simulink model "usv_twist_controller_generator_002"  (R2021b)
settings: Solver=FixedStepDiscrete  StartTime=0.0  StopTime=inf  FixedStep=twistControllerSampleTime  RelTol=1e-3  EnableMultiTasking=on
PreLoadFcn:
  | % Controller Sample Time
  | twistControllerSampleTime = 0.10;
undefined symbols (not defined in the file): DiscIntNeverNeededParam
libraries: robotlib x28, simulink x4
settings Model: Creator=altin  LastModifiedBy=altin
settings SolverCC: AllowMultiTaskInputOutput=on  ConcurrentTasks=on  PositivePriorityOrder=on  AutoInsertRateTranBlk=on
settings OptimizationCC: EnhancedBackFolding=on  PassReuseOutputArgsAs=Individual arguments  ZeroExternalMemoryAtStartup=off  ZeroInternalMemoryAtStartup=off  MaxStackSize=64  OptimizeBlockOrder=speed  DifferentSizesBufferReuse=on  OptimizationCustomize=off  EfficientTunableParamExpr=on
settings DebuggingCC: ParameterTunabilityLossMsg=error
settings HardwareCC: ProdBitPerPointer=32  ProdBitPerSizeT=32  ProdBitPerPtrDiffT=32  ProdLargestAtomicFloat=None  ProdIntDivRoundTo=Undefined  ProdEndianess=Unspecified  ProdWordSize=32  ProdHWDeviceType=Generic->Unspecified (assume 32-bit Generic)  UseEmbeddedCoderFeatures=off
settings ModelReferenceCC: ModelReferenceMinAlgLoopOccurrences=on
settings SFSimCC: MATLABDynamicMemAlloc=off
settings RTWCC: Description=Embedded Coder  SystemTargetFile=ert.tlc  HardwareBoard=Robot Operating System (ROS)  TLCOptions="-aInlineSetEventsForThisBaseRateFcn=TLC_FALSE -aSuppressMultiTaskScheduler=TLC_FALSE  -aRateBasedStepFcn=0"  TemplateMakefile=ert_default_tmf  GenerateReport=on  Toolchain=Catkin  LaunchReport=on  TargetLang=C++
settings CodeAppCC: ForceParamTrailComments=on  IgnoreCustomStorageClasses=off  OperatorAnnotations=on  SimulinkDataObjDesc=on  SFDataObjDesc=on  InsertBlockDesc=on  StateflowObjectComments=on  MATLABSourceComments=on
settings ERTTargetCC: SupportNonInlinedSFcns=on  ERTCustomFileTemplate=rostime_codertarget_file_process.tlc

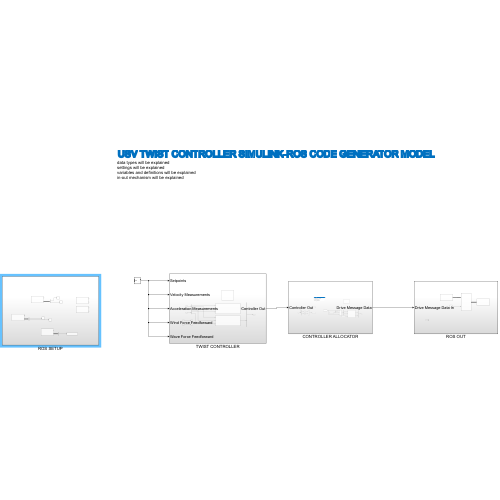
[thumbnail: Simulink's stored preview of the top-level diagram]
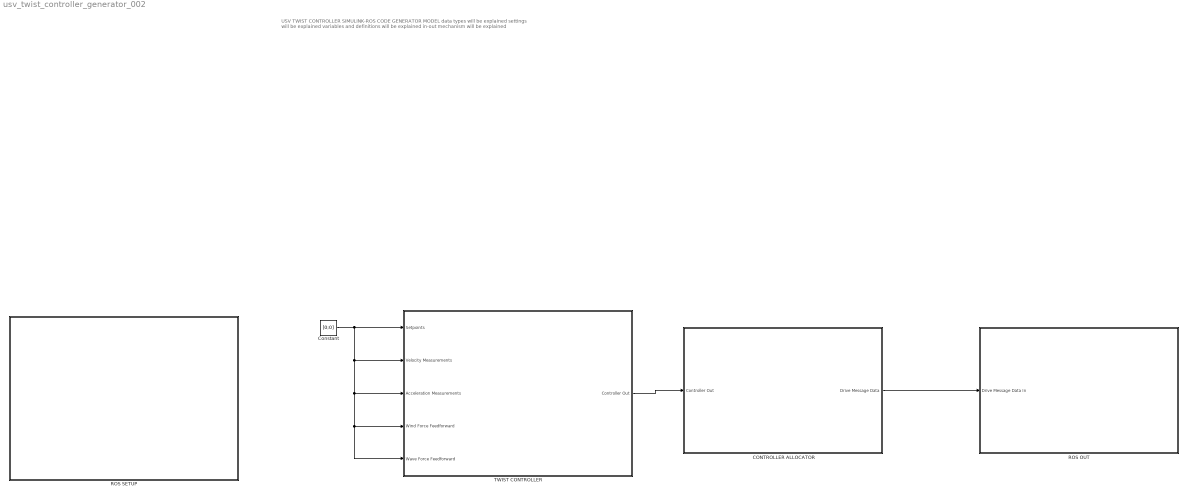
== system usv_twist_controller_generator_002 ==
  note: USV TWIST CONTROLLER SIMULINK-ROS CODE GENERATOR MODEL
      | data types will be explained
      | settings will be explained
      | variables and definitions will be explained
      | in-out mechanism will be explained
  CONTROLLER ALLOCATOR : Subsystem
  Constant : Constant  Value=[0;0]
  ROS OUT : Subsystem
  ROS SETUP : Subsystem
  TWIST CONTROLLER : Subsystem
  wires:
  TWIST CONTROLLER/1(Controller Out) -> CONTROLLER ALLOCATOR/1(Controller Out)
  CONTROLLER ALLOCATOR/1(Drive Message Data) -> ROS OUT/1(Drive Message Data In)
  Constant/1 -> TWIST CONTROLLER/1(Setpoints), TWIST CONTROLLER/2(Velocity Measurements), TWIST CONTROLLER/4(Wind Force Feedforward), TWIST CONTROLLER/5(Wave Force Feedforward), TWIST CONTROLLER/3(Acceleration Measurements)

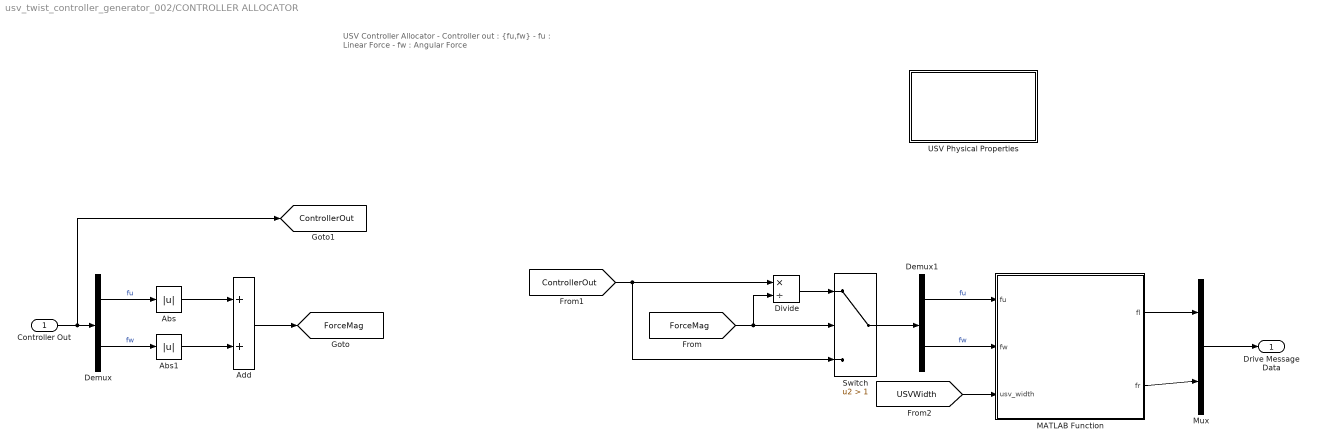
== system usv_twist_controller_generator_002/CONTROLLER ALLOCATOR ==
  note: USV Controller Allocator
      | - Controller out : {fu,fw}
      | - fu : Linear Force
      | - fw : Angular Force
  Controller Out : Inport
  Abs : Abs
  Abs1 : Abs
  Add : Sum
  Demux : Demux  Outputs=2
  Demux1 : Demux  Outputs=2
  Divide : Product  Inputs=*/
  MATLAB Function : MATLAB Function  TreatAsAtomicUnit=on
  Mux : Mux  Inputs=2
  Switch : Switch  Criteria=u2 > Threshold  Threshold=1
  USV Physical Properties : Subsystem
  Drive Message Data : Outport
  tag scope: ControllerOut=global, ForceMag=global
  wires:
  Controller Out/1 -> [ControllerOut], Demux/1
  Demux/1 -> Abs/1  "fu"
  Demux/2 -> Abs1/1  "fw"
  Abs1/1 -> Add/2
  Abs/1 -> Add/1
  Add/1 -> [ForceMag]
  [ForceMag] -> Divide/2, Switch/2
  [ControllerOut] -> Switch/3, Divide/1
  Divide/1 -> Switch/1
  Switch/1 -> Demux1/1
  [USVWidth] -> MATLAB Function/3(usv_width)
  Demux1/1 -> MATLAB Function/1(fu)  "fu"
  Demux1/2 -> MATLAB Function/2(fw)  "fw"
  MATLAB Function/1(fl) -> Mux/1
  MATLAB Function/2(fr) -> Mux/2
  Mux/1 -> Drive Message Data/1

== system usv_twist_controller_generator_002/ROS OUT ==
  Drive Message Data In : Inport
  Bus Assignment : BusAssignment  AssignedSignals=Data
  Constant : Constant  OutDataTypeStr=int32
  Motor Drive Message : robotlib/Blank Message  messageClass=Message  entityType=std_msgs/Int32  messageType=std_msgs/Int32  SampleTime=inf  legacyBusStruct=off
  USV Drive Topic : robotlib/Publish  topicSource=Specify your own  topic=/chatter2  messageType=std_msgs/Int32  legacyBusStruct=off  messageQueueLength=1
  wires:
  Motor Drive Message/1 -> Bus Assignment/1
  Constant/1 -> Bus Assignment/2
  Bus Assignment/1 -> USV Drive Topic/1

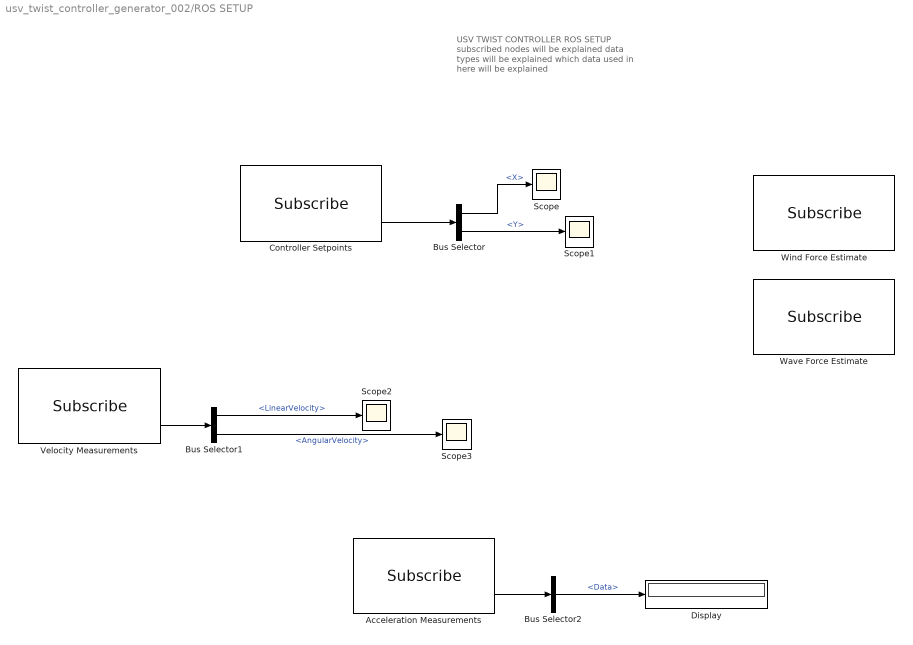
== system usv_twist_controller_generator_002/ROS SETUP ==
  note: USV TWIST CONTROLLER ROS SETUP
      | subscribed nodes will be explained
      | data types will be explained
      | which data used in here will be explained
  Acceleration Measurements : robotlib/Subscribe  topicSource=Select from ROS network  topic=/chatter  messageType=std_msgs/Int32  SampleTime=-1  legacyBusStruct=off  messageQueueLength=1
  Bus Selector : BusSelector  OutputSignals=X,Y
  Bus Selector1 : BusSelector  OutputSignals=LinearVelocity,AngularVelocity
  Bus Selector2 : BusSelector  OutputSignals=Data
  Controller Setpoints : robotlib/Subscribe  topicSource=Specify your own  topic=/gx5/nav/odom  messageType=geometry_msgs/Point  SampleTime=-1  legacyBusStruct=off  messageQueueLength=1
  Display : Display
  Scope{,1..3} (4 alike) : Scope
  Velocity Measurements : robotlib/Subscribe  topicSource=Select from ROS network  topic=/turtle1/pose  messageType=turtlesim/Pose  SampleTime=-1  legacyBusStruct=off  messageQueueLength=1
  Wave Force Estimate : robotlib/Subscribe  topicSource=Select from ROS network  topic=/my_topic  messageType=geometry_msgs/Point  SampleTime=-1  legacyBusStruct=off  messageQueueLength=1
  Wind Force Estimate : robotlib/Subscribe  topicSource=Select from ROS network  topic=/my_topic  messageType=geometry_msgs/Point  SampleTime=-1  legacyBusStruct=off  messageQueueLength=1
  wires:
  Controller Setpoints/2 -> Bus Selector/1
  Bus Selector/1 -> Scope/1  "<X>"
  Bus Selector/2 -> Scope1/1  "<Y>"
  Velocity Measurements/2 -> Bus Selector1/1
  Bus Selector1/1 -> Scope2/1  "<LinearVelocity>"
  Bus Selector1/2 -> Scope3/1  "<AngularVelocity>"
  Acceleration Measurements/2 -> Bus Selector2/1
  Bus Selector2/1 -> Display/1  "<Data>"

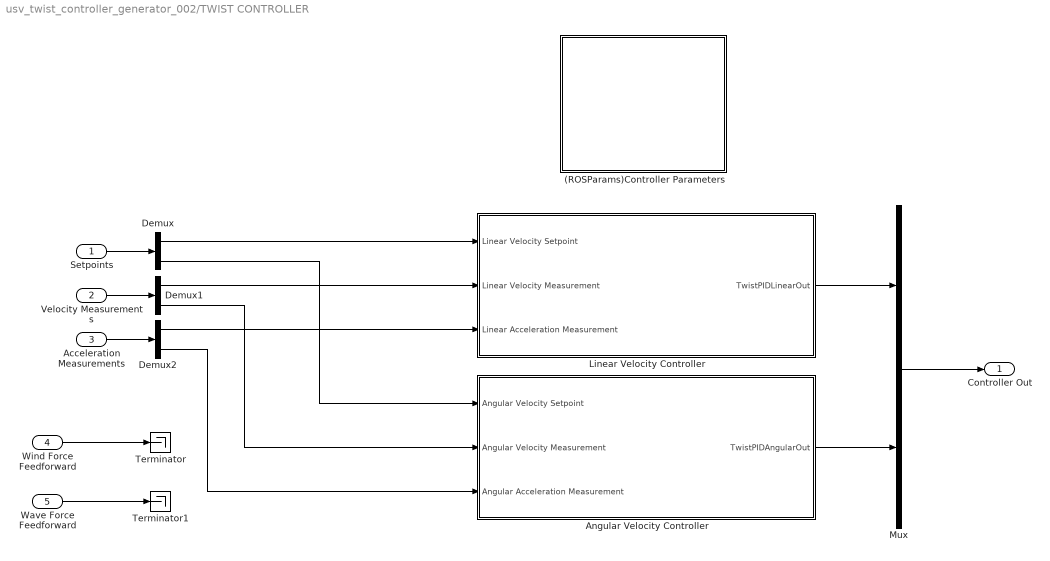
== system usv_twist_controller_generator_002/TWIST CONTROLLER ==
  Setpoints : Inport
  Velocity Measurements : Inport  Port=2
  Acceleration Measurements : Inport  Port=3
  Wind Force Feedforward : Inport  Port=4
  Wave Force Feedforward : Inport  Port=5
  (ROSParams)Controller Parameters : Subsystem
  Angular Velocity Controller : Subsystem
  Demux : Demux  Outputs=2
  Demux1 : Demux  Outputs=2
  Demux2 : Demux  Outputs=2
  Linear Velocity Controller : Subsystem
  Mux : Mux  Inputs=2
  Terminator : Terminator
  Terminator1 : Terminator
  Controller Out : Outport
  wires:
  Setpoints/1 -> Demux/1
  Demux/1 -> Linear Velocity Controller/1(Linear Velocity Setpoint)
  Demux/2 -> Angular Velocity Controller/1(Angular Velocity Setpoint)
  Wind Force Feedforward/1 -> Terminator/1
  Wave Force Feedforward/1 -> Terminator1/1
  Acceleration Measurements/1 -> Demux2/1
  Velocity Measurements/1 -> Demux1/1
  Demux1/1 -> Linear Velocity Controller/2(Linear Velocity Measurement)
  Demux1/2 -> Angular Velocity Controller/2(Angular Velocity Measurement)
  Demux2/1 -> Linear Velocity Controller/3(Linear Acceleration Measurement)
  Demux2/2 -> Angular Velocity Controller/3(Angular Acceleration Measurement)
  Linear Velocity Controller/1(TwistPIDLinearOut) -> Mux/1
  Angular Velocity Controller/1(TwistPIDAngularOut) -> Mux/2
  Mux/1 -> Controller Out/1

== system usv_twist_controller_generator_002/CONTROLLER ALLOCATOR/USV Physical Properties ==
  Twist Angular Ag : robotlib/Get Parameter  ParameterSource=Select from ROS network  ParameterName=/my_param  ParameterType=double  ParameterMaxArrayLength=16  ParameterInitialValue=0.0  SampleTime=-1  ShowErrorCodeOutput=on  ModelName=usv_twist_controller_generator_002  BlockId=ParamGet_usv_twist_controller_generator_002_280
      settings: SourceProductBaseCode=RR
  tag scope: USVWidth=global
  wires:
  Twist Angular Ag/1 -> [USVWidth]

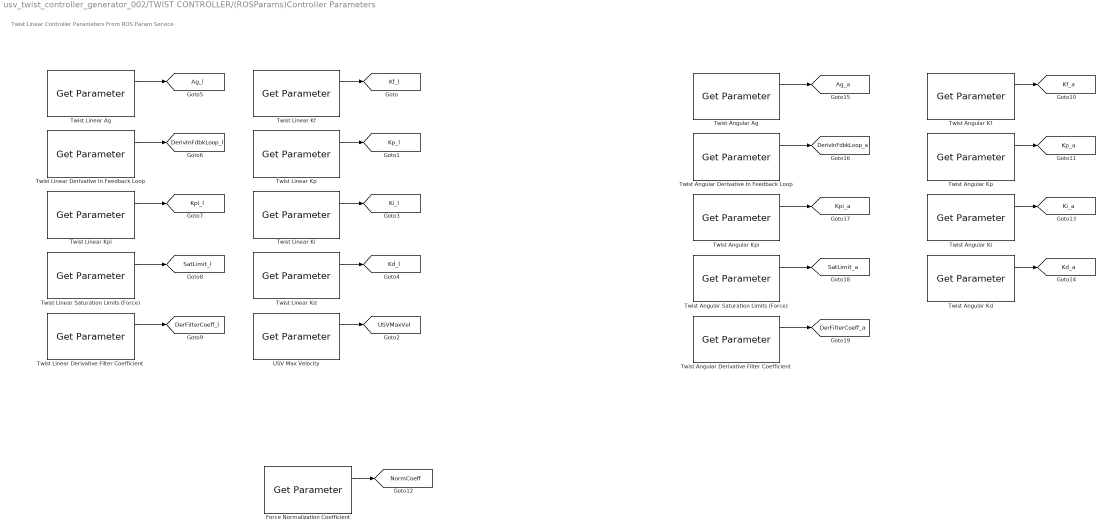
== system usv_twist_controller_generator_002/TWIST CONTROLLER/(ROSParams)Controller Parameters ==
  note: Twist Linear Controller Parameters From ROS Param Service
  Force Normalization Coefficient : robotlib/Get Parameter  ParameterSource=Select from ROS network  ParameterName=/my_param  ParameterType=double  ParameterMaxArrayLength=16  ParameterInitialValue=0.0  SampleTime=-1  ShowErrorCodeOutput=on  ModelName=usv_twist_controller_generator_002  BlockId=ParamGet_usv_twist_controller_generator_002_290
      settings: SourceProductBaseCode=RR
  Twist Angular Ag : robotlib/Get Parameter  ParameterSource=Select from ROS network  ParameterName=/my_param  ParameterType=double  ParameterMaxArrayLength=16  ParameterInitialValue=0.0  SampleTime=-1  ShowErrorCodeOutput=on  ModelName=usv_twist_controller_generator_002  BlockId=ParamGet_usv_twist_controller_generator_002_169
      settings: SourceProductBaseCode=RR
  Twist Angular Derivative Filter Coefficient : robotlib/Get Parameter  ParameterSource=Select from ROS network  ParameterName=/my_param  ParameterType=double  ParameterMaxArrayLength=16  ParameterInitialValue=0.0  SampleTime=-1  ShowErrorCodeOutput=on  ModelName=usv_twist_controller_generator_002  BlockId=ParamGet_usv_twist_controller_generator_002_170
      settings: SourceProductBaseCode=RR
  Twist Angular Derivative In Feedback Loop : robotlib/Get Parameter  ParameterSource=Select from ROS network  ParameterName=/my_param  ParameterType=double  ParameterMaxArrayLength=16  ParameterInitialValue=0.0  SampleTime=-1  ShowErrorCodeOutput=on  ModelName=usv_twist_controller_generator_002  BlockId=ParamGet_usv_twist_controller_generator_002_171
      settings: SourceProductBaseCode=RR
  Twist Angular Kd : robotlib/Get Parameter  ParameterSource=Select from ROS network  ParameterName=/my_param  ParameterType=double  ParameterMaxArrayLength=16  ParameterInitialValue=0.0  SampleTime=-1  ShowErrorCodeOutput=on  ModelName=usv_twist_controller_generator_002  BlockId=ParamGet_usv_twist_controller_generator_002_172
      settings: SourceProductBaseCode=RR
  Twist Angular Kf : robotlib/Get Parameter  ParameterSource=Select from ROS network  ParameterName=/my_param  ParameterType=double  ParameterMaxArrayLength=16  ParameterInitialValue=0.0  SampleTime=-1  ShowErrorCodeOutput=on  ModelName=usv_twist_controller_generator_002  BlockId=ParamGet_usv_twist_controller_generator_002_173
      settings: SourceProductBaseCode=RR
  Twist Angular Ki : robotlib/Get Parameter  ParameterSource=Select from ROS network  ParameterName=/my_param  ParameterType=double  ParameterMaxArrayLength=16  ParameterInitialValue=0.0  SampleTime=-1  ShowErrorCodeOutput=on  ModelName=usv_twist_controller_generator_002  BlockId=ParamGet_usv_twist_controller_generator_002_174
      settings: SourceProductBaseCode=RR
  Twist Angular Kp : robotlib/Get Parameter  ParameterSource=Select from ROS network  ParameterName=/my_param  ParameterType=double  ParameterMaxArrayLength=16  ParameterInitialValue=0.0  SampleTime=-1  ShowErrorCodeOutput=on  ModelName=usv_twist_controller_generator_002  BlockId=ParamGet_usv_twist_controller_generator_002_175
      settings: SourceProductBaseCode=RR
  Twist Angular Kpi : robotlib/Get Parameter  ParameterSource=Select from ROS network  ParameterName=/my_param  ParameterType=double  ParameterMaxArrayLength=16  ParameterInitialValue=0.0  SampleTime=-1  ShowErrorCodeOutput=on  ModelName=usv_twist_controller_generator_002  BlockId=ParamGet_usv_twist_controller_generator_002_176
      settings: SourceProductBaseCode=RR
  Twist Angular Saturation Limits (Force) : robotlib/Get Parameter  ParameterSource=Select from ROS network  ParameterName=/my_param  ParameterType=double  ParameterMaxArrayLength=16  ParameterInitialValue=0.0  SampleTime=-1  ShowErrorCodeOutput=on  ModelName=usv_twist_controller_generator_002  BlockId=ParamGet_usv_twist_controller_generator_002_177
      settings: SourceProductBaseCode=RR
  Twist Linear Ag : robotlib/Get Parameter  ParameterSource=Select from ROS network  ParameterName=/my_param  ParameterType=double  ParameterMaxArrayLength=16  ParameterInitialValue=0.0  SampleTime=-1  ShowErrorCodeOutput=on  ModelName=usv_twist_controller_generator_002  BlockId=ParamGet_usv_twist_controller_generator_002_9
      settings: SourceProductBaseCode=RR
  Twist Linear Derivative Filter Coefficient : robotlib/Get Parameter  ParameterSource=Select from ROS network  ParameterName=/my_param  ParameterType=double  ParameterMaxArrayLength=16  ParameterInitialValue=0.0  SampleTime=-1  ShowErrorCodeOutput=on  ModelName=usv_twist_controller_generator_002  BlockId=ParamGet_usv_twist_controller_generator_002_50
      settings: SourceProductBaseCode=RR
  Twist Linear Derivative In Feedback Loop : robotlib/Get Parameter  ParameterSource=Select from ROS network  ParameterName=/my_param  ParameterType=double  ParameterMaxArrayLength=16  ParameterInitialValue=0.0  SampleTime=-1  ShowErrorCodeOutput=on  ModelName=usv_twist_controller_generator_002  BlockId=ParamGet_usv_twist_controller_generator_002_10
      settings: SourceProductBaseCode=RR
  Twist Linear Kd : robotlib/Get Parameter  ParameterSource=Select from ROS network  ParameterName=/my_param  ParameterType=double  ParameterMaxArrayLength=16  ParameterInitialValue=0.0  SampleTime=-1  ShowErrorCodeOutput=on  ModelName=usv_twist_controller_generator_002  BlockId=ParamGet_usv_twist_controller_generator_002_8
      settings: SourceProductBaseCode=RR
  Twist Linear Kf : robotlib/Get Parameter  ParameterSource=Select from ROS network  ParameterName=/my_param  ParameterType=double  ParameterMaxArrayLength=16  ParameterInitialValue=0.0  SampleTime=-1  ShowErrorCodeOutput=on  ModelName=usv_twist_controller_generator_002  BlockId=ParamGet_usv_twist_controller_generator_002_11
      settings: SourceProductBaseCode=RR
  Twist Linear Ki : robotlib/Get Parameter  ParameterSource=Select from ROS network  ParameterName=/my_param  ParameterType=double  ParameterMaxArrayLength=16  ParameterInitialValue=0.0  SampleTime=-1  ShowErrorCodeOutput=on  ModelName=usv_twist_controller_generator_002  BlockId=ParamGet_usv_twist_controller_generator_002_7
      settings: SourceProductBaseCode=RR
  Twist Linear Kp : robotlib/Get Parameter  ParameterSource=Select from ROS network  ParameterName=/my_param  ParameterType=double  ParameterMaxArrayLength=16  ParameterInitialValue=0.0  SampleTime=-1  ShowErrorCodeOutput=on  ModelName=usv_twist_controller_generator_002  BlockId=ParamGet_usv_twist_controller_generator_002_3
      settings: SourceProductBaseCode=RR
  Twist Linear Kpi : robotlib/Get Parameter  ParameterSource=Select from ROS network  ParameterName=/my_param  ParameterType=double  ParameterMaxArrayLength=16  ParameterInitialValue=0.0  SampleTime=-1  ShowErrorCodeOutput=on  ModelName=usv_twist_controller_generator_002  BlockId=ParamGet_usv_twist_controller_generator_002_12
      settings: SourceProductBaseCode=RR
  Twist Linear Saturation Limits (Force) : robotlib/Get Parameter  ParameterSource=Select from ROS network  ParameterName=/my_param  ParameterType=double  ParameterMaxArrayLength=16  ParameterInitialValue=0.0  SampleTime=-1  ShowErrorCodeOutput=on  ModelName=usv_twist_controller_generator_002  BlockId=ParamGet_usv_twist_controller_generator_002_13
      settings: SourceProductBaseCode=RR
  USV Max Velocity : robotlib/Get Parameter  ParameterSource=Select from ROS network  ParameterName=/my_param  ParameterType=double  ParameterMaxArrayLength=16  ParameterInitialValue=0.0  SampleTime=-1  ShowErrorCodeOutput=on  ModelName=usv_twist_controller_generator_002  BlockId=ParamGet_usv_twist_controller_generator_002_21
      settings: SourceProductBaseCode=RR
  tag scope: Ag_a=global, Ag_l=global, DerFilterCoeff_a=global, DerFilterCoeff_l=global, DerivInFdbkLoop_a=global, DerivInFdbkLoop_l=global, Kd_a=global, Kd_l=global, Kf_a=global, Kf_l=global, Ki_a=global, Ki_l=global, Kp_a=global, Kp_l=global, Kpi_a=global, Kpi_l=global, NormCoeff=global, SatLimit_a=global, SatLimit_l=global, USVMaxVel=global
  wires:
  Twist Linear Kf/1 -> [Kf_l]
  Twist Linear Kp/1 -> [Kp_l]
  Twist Linear Ki/1 -> [Ki_l]
  Twist Linear Kd/1 -> [Kd_l]
  USV Max Velocity/1 -> [USVMaxVel]
  Twist Linear Ag/1 -> [Ag_l]
  Twist Linear Derivative In Feedback Loop/1 -> [DerivInFdbkLoop_l]
  Twist Linear Kpi/1 -> [Kpi_l]
  Twist Linear Saturation Limits (Force)/1 -> [SatLimit_l]
  Twist Linear Derivative Filter Coefficient/1 -> [DerFilterCoeff_l]
  Twist Angular Saturation Limits (Force)/1 -> [SatLimit_a]
  Twist Angular Ag/1 -> [Ag_a]
  Twist Angular Kpi/1 -> [Kpi_a]
  Twist Angular Kf/1 -> [Kf_a]
  Twist Angular Derivative Filter Coefficient/1 -> [DerFilterCoeff_a]
  Twist Angular Ki/1 -> [Ki_a]
  Twist Angular Kp/1 -> [Kp_a]
  Twist Angular Kd/1 -> [Kd_a]
  Twist Angular Derivative In Feedback Loop/1 -> [DerivInFdbkLoop_a]
  Force Normalization Coefficient/1 -> [NormCoeff]

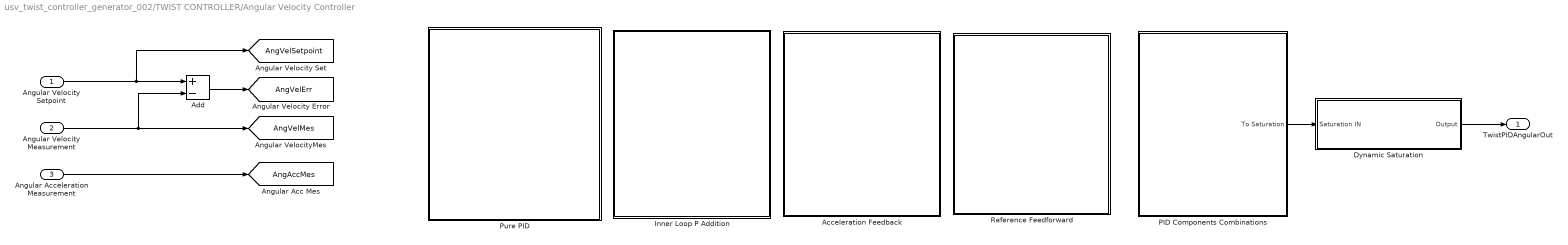
== system usv_twist_controller_generator_002/TWIST CONTROLLER/Angular Velocity Controller ==
  Angular Velocity Setpoint : Inport
  Angular Velocity Measurement : Inport  Port=2
  Angular Acceleration Measurement : Inport  Port=3
  Acceleration Feedback : Subsystem
  Add : Sum  Inputs=+-
  Dynamic Saturation : Subsystem
  Inner Loop P Addition : Subsystem
  PID Components Combinations : Subsystem
  Pure PID : Subsystem
  Reference Feedforward : Subsystem
  TwistPIDAngularOut : Outport
  tag scope: AngAccMes=global, AngVelErr=global, AngVelMes=global, AngVelSetpoint=global
  wires:
  PID Components Combinations/1(To Saturation) -> Dynamic Saturation/1(Saturation IN)
  Angular Acceleration Measurement/1 -> [AngAccMes]
  Angular Velocity Measurement/1 -> [AngVelMes], Add/2
  Angular Velocity Setpoint/1 -> [AngVelSetpoint], Add/1
  Add/1 -> [AngVelErr]
  Dynamic Saturation/1(Output) -> TwistPIDAngularOut/1

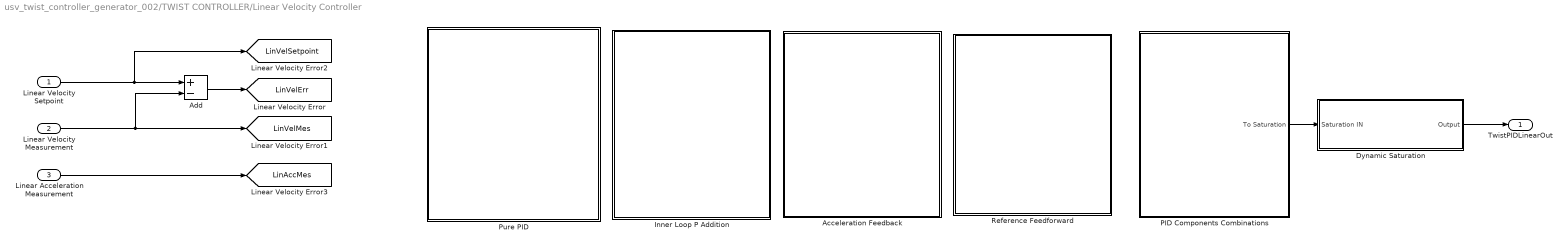
== system usv_twist_controller_generator_002/TWIST CONTROLLER/Linear Velocity Controller ==
  Linear Velocity Setpoint : Inport
  Linear Velocity Measurement : Inport  Port=2
  Linear Acceleration Measurement : Inport  Port=3
  Acceleration Feedback : Subsystem
  Add : Sum  Inputs=+-
  Dynamic Saturation : Subsystem
  Inner Loop P Addition : Subsystem
  PID Components Combinations : Subsystem
  Pure PID : Subsystem
  Reference Feedforward : Subsystem
  TwistPIDLinearOut : Outport
  tag scope: LinAccMes=global, LinVelErr=global, LinVelMes=global, LinVelSetpoint=global
  wires:
  Linear Velocity Setpoint/1 -> [LinVelSetpoint], Add/1
  Linear Velocity Measurement/1 -> [LinVelMes], Add/2
  Add/1 -> [LinVelErr]
  Linear Acceleration Measurement/1 -> [LinAccMes]
  Dynamic Saturation/1(Output) -> TwistPIDLinearOut/1
  PID Components Combinations/1(To Saturation) -> Dynamic Saturation/1(Saturation IN)

== system usv_twist_controller_generator_002/TWIST CONTROLLER/Angular Velocity Controller/Acceleration Feedback ==
  Product : Product
  tag scope: AccFdbkOut_a=global
  wires:
  [AngAccMes] -> Product/1
  [Ag_a] -> Product/2
  Product/1 -> [AccFdbkOut_a]

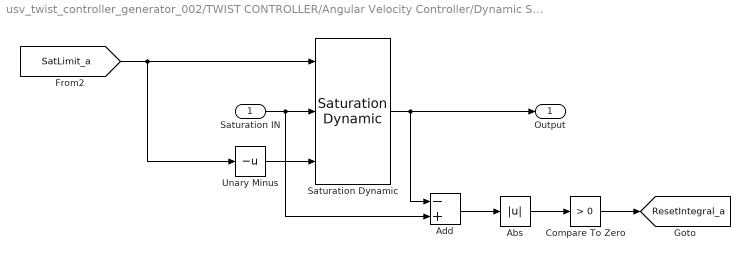
== system usv_twist_controller_generator_002/TWIST CONTROLLER/Angular Velocity Controller/Dynamic Saturation ==
  Saturation IN : Inport
  Abs : Abs
  Add : Sum  Inputs=-+
  Compare To Zero : simulink/Logic and Bit Operations/Compare To Zero  relop=>  OutDataTypeStr=boolean
  Saturation Dynamic : simulink/Discontinuities/Saturation Dynamic  OutMin=[]  OutMax=[]  OutDataTypeStr=Inherit: Same as second input  OutDataType=fixdt(1, 16)  OutScaling=2^-10  DoSatur=off
  Unary Minus : UnaryMinus
  Output : Outport
  tag scope: ResetIntegral_a=global
  wires:
  Unary Minus/1 -> Saturation Dynamic/3
  [SatLimit_a] -> Saturation Dynamic/1, Unary Minus/1
  Saturation IN/1 -> Add/2, Saturation Dynamic/2
  Saturation Dynamic/1 -> Output/1, Add/1
  Add/1 -> Abs/1
  Abs/1 -> Compare To Zero/1
  Compare To Zero/1 -> [ResetIntegral_a]

== system usv_twist_controller_generator_002/TWIST CONTROLLER/Angular Velocity Controller/Inner Loop P Addition ==
  note: Inner-Loop P Controller
  Add3 : Sum  Inputs=+-
  Product4 : Product
  tag scope: PIDWInnerLoopP_a=global
  wires:
  [AngVelMes] -> Add3/2
  [Kpi_a] -> Product4/2
  Product4/1 -> [PIDWInnerLoopP_a]
  [PIDOut_a] -> Add3/1
  Add3/1 -> Product4/1

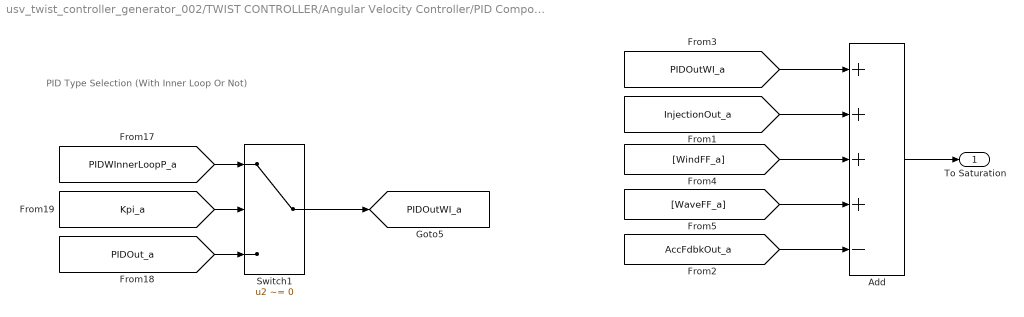
== system usv_twist_controller_generator_002/TWIST CONTROLLER/Angular Velocity Controller/PID Components Combinations ==
  note: PID Type Selection (With Inner Loop Or Not)
  Add : Sum  Inputs=++++-
  Switch1 : Switch  Criteria=u2 ~= 0
  To Saturation : Outport
  tag scope: PIDOutWI_a=global
  wires:
  [PIDOut_a] -> Switch1/3
  [PIDWInnerLoopP_a] -> Switch1/1
  Switch1/1 -> [PIDOutWI_a]
  [Kpi_a] -> Switch1/2
  [AccFdbkOut_a] -> Add/5
  [WaveFF_a] -> Add/4
  [WindFF_a] -> Add/3
  [InjectionOut_a] -> Add/2
  [PIDOutWI_a] -> Add/1
  Add/1 -> To Saturation/1

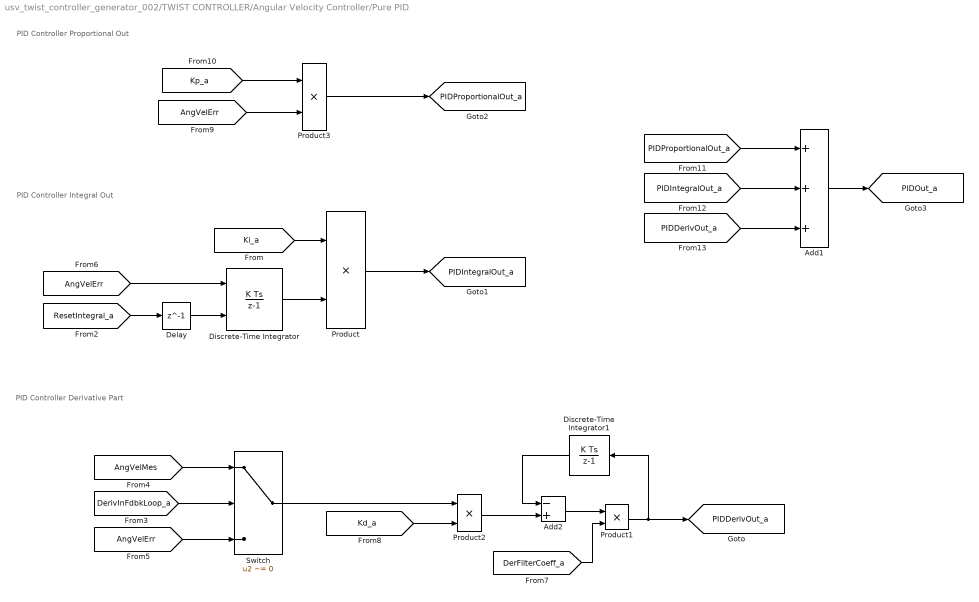
== system usv_twist_controller_generator_002/TWIST CONTROLLER/Angular Velocity Controller/Pure PID ==
  note: PID Controller Derivative Part
  note: PID Controller Integral Out
  note: PID Controller Proportional Out
  Add1 : Sum  Inputs=+++
  Add2 : Sum  Inputs=-+
  Delay : Delay  DelayLength=1
  Discrete-Time Integrator : DiscreteIntegrator  ExternalReset=level  SampleTime=twistControllerSampleTime  ICPrevOutput=DiscIntNeverNeededParam  ICPrevScaledInput=DiscIntNeverNeededParam
  Discrete-Time Integrator1 : DiscreteIntegrator  SampleTime=twistControllerSampleTime  ICPrevOutput=DiscIntNeverNeededParam  ICPrevScaledInput=DiscIntNeverNeededParam
  Product{,1..3} (4 alike) : Product
  Switch : Switch  Criteria=u2 ~= 0
  tag scope: PIDDerivOut_a=global, PIDIntegralOut_a=global, PIDOut_a=global, PIDProportionalOut_a=global
  wires:
  Product/1 -> [PIDIntegralOut_a]
  Product3/1 -> [PIDProportionalOut_a]
  Product1/1 -> [PIDDerivOut_a], Discrete-Time Integrator1/1
  [DerivInFdbkLoop_a] -> Switch/2
  [AngVelMes] -> Switch/1
  Product2/1 -> Add2/2
  [Kd_a] -> Product2/2
  Switch/1 -> Product2/1
  [Kp_a] -> Product3/1
  [AngVelErr] -> Product3/2
  [DerFilterCoeff_a] -> Product1/2
  Discrete-Time Integrator/1 -> Product/2
  Add2/1 -> Product1/1
  [AngVelErr] -> Discrete-Time Integrator/1
  [Ki_a] -> Product/1
  [AngVelErr] -> Switch/3
  Discrete-Time Integrator1/1 -> Add2/1
  [PIDIntegralOut_a] -> Add1/2
  Add1/1 -> [PIDOut_a]
  [PIDDerivOut_a] -> Add1/3
  [PIDProportionalOut_a] -> Add1/1
  [ResetIntegral_a] -> Delay/1
  Delay/1 -> Discrete-Time Integrator/2

== system usv_twist_controller_generator_002/TWIST CONTROLLER/Angular Velocity Controller/Reference Feedforward ==
  note: Reference Injection (Velocity Feedforward)
  Product5 : Product
  tag scope: InjectionOut_a=global
  wires:
  [AngVelSetpoint] -> Product5/1
  Product5/1 -> [InjectionOut_a]
  [Kf_a] -> Product5/2

== system usv_twist_controller_generator_002/TWIST CONTROLLER/Linear Velocity Controller/Acceleration Feedback ==
  Product : Product
  tag scope: AccFdbkOut_l=global
  wires:
  [LinAccMes] -> Product/1
  [Ag_l] -> Product/2
  Product/1 -> [AccFdbkOut_l]

== system usv_twist_controller_generator_002/TWIST CONTROLLER/Linear Velocity Controller/Dynamic Saturation ==
  Saturation IN : Inport
  Abs : Abs
  Add : Sum  Inputs=-+
  Compare To Zero : simulink/Logic and Bit Operations/Compare To Zero  relop=>  OutDataTypeStr=boolean
  Saturation Dynamic : simulink/Discontinuities/Saturation Dynamic  OutMin=[]  OutMax=[]  OutDataTypeStr=Inherit: Same as second input  OutDataType=fixdt(1, 16)  OutScaling=2^-10  DoSatur=off
  Unary Minus : UnaryMinus
  Output : Outport
  tag scope: ResetIntegral_l=global
  wires:
  Unary Minus/1 -> Saturation Dynamic/3
  [SatLimit_l] -> Saturation Dynamic/1, Unary Minus/1
  Saturation IN/1 -> Add/2, Saturation Dynamic/2
  Saturation Dynamic/1 -> Output/1, Add/1
  Add/1 -> Abs/1
  Abs/1 -> Compare To Zero/1
  Compare To Zero/1 -> [ResetIntegral_l]

== system usv_twist_controller_generator_002/TWIST CONTROLLER/Linear Velocity Controller/Inner Loop P Addition ==
  note: Inner-Loop P Controller
  Add3 : Sum  Inputs=+-
  Product4 : Product
  tag scope: PIDWInnerLoopP_l=global
  wires:
  [LinVelMes] -> Add3/2
  [Kpi_l] -> Product4/2
  Product4/1 -> [PIDWInnerLoopP_l]
  [PIDOut_l] -> Add3/1
  Add3/1 -> Product4/1

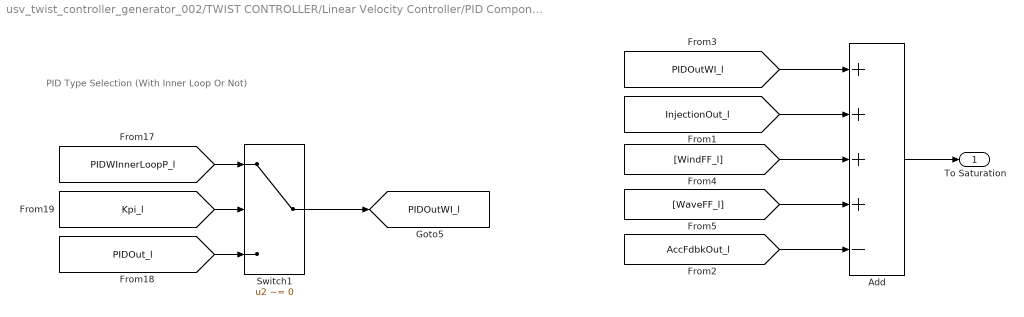
== system usv_twist_controller_generator_002/TWIST CONTROLLER/Linear Velocity Controller/PID Components Combinations ==
  note: PID Type Selection (With Inner Loop Or Not)
  Add : Sum  Inputs=++++-
  Switch1 : Switch  Criteria=u2 ~= 0
  To Saturation : Outport
  tag scope: PIDOutWI_l=global
  wires:
  [PIDOut_l] -> Switch1/3
  [PIDWInnerLoopP_l] -> Switch1/1
  Switch1/1 -> [PIDOutWI_l]
  [Kpi_l] -> Switch1/2
  [AccFdbkOut_l] -> Add/5
  [WaveFF_l] -> Add/4
  [WindFF_l] -> Add/3
  [InjectionOut_l] -> Add/2
  [PIDOutWI_l] -> Add/1
  Add/1 -> To Saturation/1

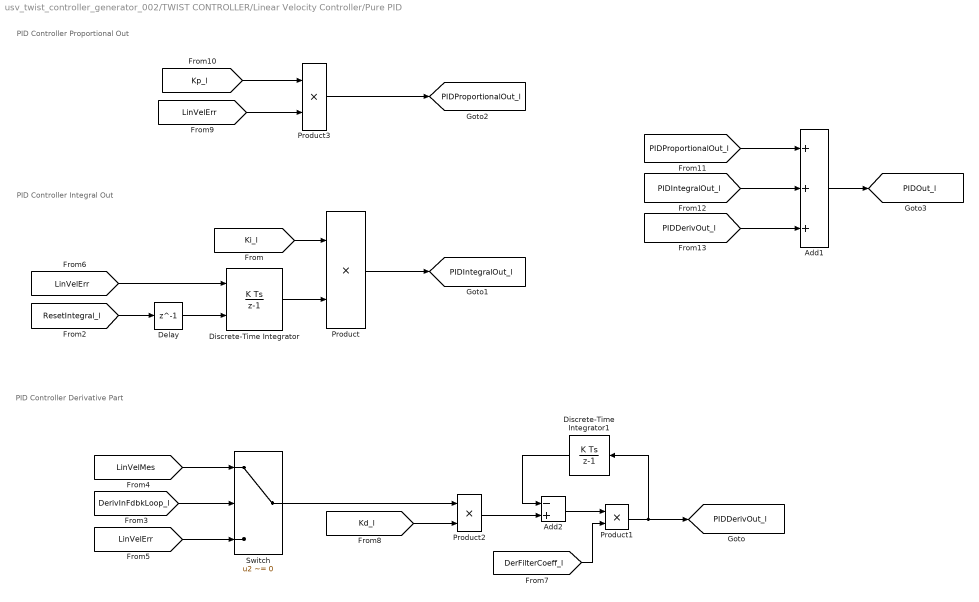
== system usv_twist_controller_generator_002/TWIST CONTROLLER/Linear Velocity Controller/Pure PID ==
  note: PID Controller Derivative Part
  note: PID Controller Integral Out
  note: PID Controller Proportional Out
  Add1 : Sum  Inputs=+++
  Add2 : Sum  Inputs=-+
  Delay : Delay  DelayLength=1
  Discrete-Time Integrator : DiscreteIntegrator  ExternalReset=level  SampleTime=twistControllerSampleTime  ICPrevOutput=DiscIntNeverNeededParam  ICPrevScaledInput=DiscIntNeverNeededParam
  Discrete-Time Integrator1 : DiscreteIntegrator  SampleTime=twistControllerSampleTime  ICPrevOutput=DiscIntNeverNeededParam  ICPrevScaledInput=DiscIntNeverNeededParam
  Product{,1..3} (4 alike) : Product
  Switch : Switch  Criteria=u2 ~= 0
  tag scope: PIDDerivOut_l=global, PIDIntegralOut_l=global, PIDOut_l=global, PIDProportionalOut_l=global
  wires:
  Product/1 -> [PIDIntegralOut_l]
  Product3/1 -> [PIDProportionalOut_l]
  Product1/1 -> [PIDDerivOut_l], Discrete-Time Integrator1/1
  [DerivInFdbkLoop_l] -> Switch/2
  [LinVelMes] -> Switch/1
  Product2/1 -> Add2/2
  [Kd_l] -> Product2/2
  Switch/1 -> Product2/1
  [Kp_l] -> Product3/1
  [LinVelErr] -> Product3/2
  [DerFilterCoeff_l] -> Product1/2
  Discrete-Time Integrator/1 -> Product/2
  Add2/1 -> Product1/1
  [LinVelErr] -> Discrete-Time Integrator/1
  [Ki_l] -> Product/1
  [LinVelErr] -> Switch/3
  Discrete-Time Integrator1/1 -> Add2/1
  [PIDIntegralOut_l] -> Add1/2
  Add1/1 -> [PIDOut_l]
  [PIDDerivOut_l] -> Add1/3
  [PIDProportionalOut_l] -> Add1/1
  [ResetIntegral_l] -> Delay/1
  Delay/1 -> Discrete-Time Integrator/2

== system usv_twist_controller_generator_002/TWIST CONTROLLER/Linear Velocity Controller/Reference Feedforward ==
  note: Reference Injection (Velocity Feedforward)
  Product5 : Product
  tag scope: InjectionOut_l=global
  wires:
  [LinVelSetpoint] -> Product5/1
  Product5/1 -> [InjectionOut_l]
  [Kf_l] -> Product5/2

== matlab function usv_twist_controller_generator_002/CONTROLLER ALLOCATOR/MATLAB Function ==
  data: fu input; fl output; fw input; fr output; usv_width input
function [fl,fr] = controller_allocator(fu,fw,usv_width)

% Calculate the right and left motor necessary forces
fr = (fu/2)+(fw/usv_width);
fl = (fu/2)-(fw/usv_width);
